simulink model "modelClosedLoop"  (R2019b)
settings: Solver=VariableStepAuto  StartTime=0.0  StopTime=Tsim  RelTol=1e-3
values from neighbouring files (symbols this model uses):
  vx = 2.0    (= 2)    [init_sim.m]
  X0 = zeros(7, 1)    [init_sim.m]
undefined symbols (not defined in the file or in its folder): Controlador, controllerGainsCurve, params, Ts_guidance, useCourse, userParameters, wps
settings Model: Creator=renan  LastModifiedBy=renan

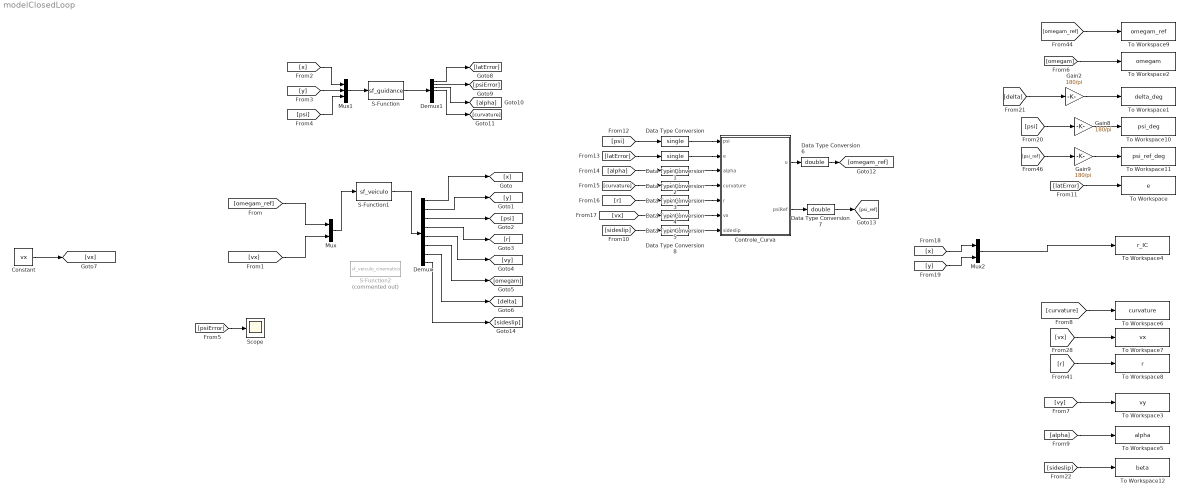
== system modelClosedLoop ==
  Constant : Constant  Value=vx
  Controle_Curva : Subsystem  TreatAsAtomicUnit=on
  Data Type Conversion{,1..5,8} (7 alike) : DataTypeConversion  OutDataTypeStr=single
  Data Type Conversion6 : DataTypeConversion  OutDataTypeStr=double
  Data Type Conversion7 : DataTypeConversion  OutDataTypeStr=double
  Demux : Demux  Outputs=8
  Demux1 : Demux  Outputs=7
  Gain2 : Gain  Gain=180/pi
  Gain8 : Gain  Gain=180/pi
  Gain9 : Gain  Gain=180/pi
  Mux : Mux  Inputs=2
  Mux1 : Mux  Inputs=3
  Mux2 : Mux  Inputs=2
  S-Function : S-Function  FunctionName=sf_guidance  Parameters=wps,Ts_guidance  SFunctionDeploymentMode=off  EnableBusSupport=off
  S-Function1 : S-Function  FunctionName=sf_veiculo  Parameters=X0,params  SFunctionDeploymentMode=off  EnableBusSupport=off
  S-Function2 : S-Function  Commented=on  FunctionName=sf_veiculo_cinematico  Parameters=X0,params  SFunctionDeploymentMode=off  EnableBusSupport=off
  Scope : Scope
  To Workspace : ToWorkspace  VariableName=e  SaveFormat=Structure With Time  SampleTime=0.01
  To Workspace1 : ToWorkspace  VariableName=delta_deg  SaveFormat=Structure With Time  SampleTime=0.01
  To Workspace10 : ToWorkspace  VariableName=psi_deg  SaveFormat=Structure With Time  SampleTime=0.01
  To Workspace11 : ToWorkspace  VariableName=psi_ref_deg  SaveFormat=Structure With Time  SampleTime=0.01
  To Workspace12 : ToWorkspace  VariableName=beta  SaveFormat=Structure With Time  SampleTime=0.01
  To Workspace2 : ToWorkspace  VariableName=omegam  SaveFormat=Structure With Time  SampleTime=0.01
  To Workspace3 : ToWorkspace  VariableName=vy  SaveFormat=Structure With Time  SampleTime=0.01
  To Workspace4 : ToWorkspace  VariableName=r_IC  SaveFormat=Structure With Time  SampleTime=0.01
  To Workspace5 : ToWorkspace  VariableName=alpha  SaveFormat=Structure With Time  SampleTime=0.01
  To Workspace6 : ToWorkspace  VariableName=curvature  SaveFormat=Structure With Time  SampleTime=0.01
  To Workspace7 : ToWorkspace  VariableName=vx  SaveFormat=Structure With Time  SampleTime=0.01
  To Workspace8 : ToWorkspace  VariableName=r  SaveFormat=Structure With Time  SampleTime=0.01
  To Workspace9 : ToWorkspace  VariableName=omegam_ref  SaveFormat=Structure With Time  SampleTime=0.01
  wires:
  Mux/1 -> S-Function1/1
  [omegam_ref] -> Mux/1
  [vx] -> Mux/2
  S-Function1/1 -> Demux/1
  Demux/1 -> [x]
  Demux/2 -> [y]
  Demux/3 -> [psi]
  Demux/4 -> [r]
  Demux/5 -> [vy]
  Demux/6 -> [omegam]
  Demux/7 -> [delta]
  Constant/1 -> [vx]
  [x] -> Mux1/1
  [y] -> Mux1/2
  Mux1/1 -> S-Function/1
  [psi] -> Mux1/3
  S-Function/1 -> Demux1/1
  Demux1/1 -> [latError]
  Demux1/2 -> [psiError]
  Demux1/3 -> [alpha]
  Demux1/4 -> [curvature]
  [latError] -> Data Type Conversion1/1
  [alpha] -> Data Type Conversion2/1
  [curvature] -> Data Type Conversion3/1
  [r] -> Data Type Conversion4/1
  [vx] -> Data Type Conversion5/1
  Controle_Curva/1(u) -> Data Type Conversion6/1
  Data Type Conversion/1 -> Controle_Curva/1(psi)
  Data Type Conversion1/1 -> Controle_Curva/2(e)
  Data Type Conversion2/1 -> Controle_Curva/3(alpha)
  Data Type Conversion3/1 -> Controle_Curva/4(curvature)
  Data Type Conversion4/1 -> Controle_Curva/5(r)
  Data Type Conversion5/1 -> Controle_Curva/6(vx)
  Data Type Conversion6/1 -> [omegam_ref]
  [curvature] -> To Workspace6/1
  Gain8/1 -> To Workspace10/1
  [latError] -> To Workspace/1
  [psi] -> Gain8/1
  Gain2/1 -> To Workspace1/1
  Gain9/1 -> To Workspace11/1
  [psi_ref] -> Gain9/1
  [omegam] -> To Workspace2/1
  [r] -> To Workspace8/1
  [omegam_ref] -> To Workspace9/1
  [vx] -> To Workspace7/1
  Mux2/1 -> To Workspace4/1
  [delta] -> Gain2/1
  Controle_Curva/2(psiRef) -> Data Type Conversion7/1
  Data Type Conversion7/1 -> [psi_ref]
  [x] -> Mux2/1
  [y] -> Mux2/2
  [psiError] -> Scope/1
  [vy] -> To Workspace3/1
  [alpha] -> To Workspace5/1
  Demux/8 -> [sideslip]
  [psi] -> Data Type Conversion/1
  [sideslip] -> Data Type Conversion8/1
  Data Type Conversion8/1 -> Controle_Curva/7(sideslip)
  [sideslip] -> To Workspace12/1

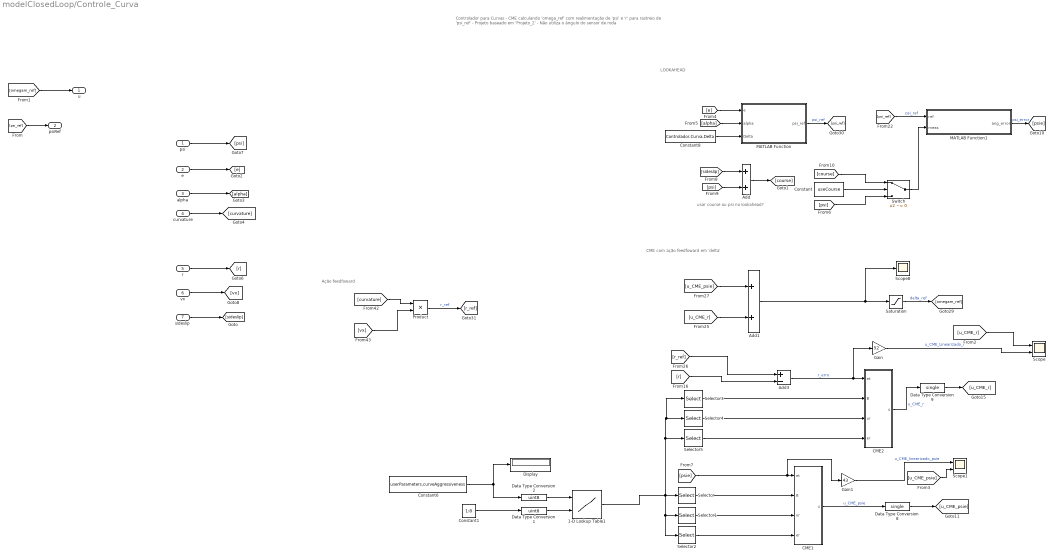
== system modelClosedLoop/Controle_Curva ==
  note: usar course ou psi no lookahead?
  note: Controlador para Curvas
      |
      | - CME calculando 'omega_ref' com realimentação de 'psi' e 'r' para rastreio de 'psi_ref'
      | - Projeto baseado em 'Projeto_2'
      | - Não utiliza o ângulo do sensor de roda
  note: LOOKAHEAD
  note: CME com ação feedfoward em 'delta'
  note: Ação feedfoward
  psi : Inport  OutDataTypeStr=single  PortDimensions=1
  e : Inport  Port=2  OutDataTypeStr=single  PortDimensions=1
  alpha : Inport  Port=3  OutDataTypeStr=single  PortDimensions=1
  curvature : Inport  Port=4  OutDataTypeStr=single  PortDimensions=1
  r : Inport  Port=5  OutDataTypeStr=single  PortDimensions=1
  vx : Inport  Port=6  OutDataTypeStr=single  PortDimensions=1
  sideslip : Inport  Port=7
  1-D Lookup Table1 : Lookup_n-D  BreakpointsForDimension1=uint8(1:7)  BreakpointsForDimension2=uint8(1:8)  IndexSearchMethod=Linear search  BeginIndexSearchUsingPreviousIndexResult=on  Table=controllerGainsCurve  ExtrapMethod=Clip  UseLastTableValue=on  InternalRulePriority=Speed  OutDataTypeStr=single  RndMeth=Simplest  InputSameDT=on
  Add : Sum
  Add1 : Sum
  Add3 : Sum  Inputs=+-
  CME1 : MATLAB Function  TreatAsAtomicUnit=on
  CME2 : MATLAB Function  TreatAsAtomicUnit=on
  Constant : Constant  Value=useCourse
  Constant1 : Constant  Value=1:8
  Constant6 : Constant  Value=userParameters.curveAggressiveness
  Constant8 : Constant  Value=Controlador.Curva.Delta  SampleTime=-1
  Data Type Conversion1 : DataTypeConversion  OutDataTypeStr=uint8
  Data Type Conversion2 : DataTypeConversion  OutDataTypeStr=uint8
  Data Type Conversion8 : DataTypeConversion  OutDataTypeStr=single
  Data Type Conversion9 : DataTypeConversion  OutDataTypeStr=single
  Display : Display
  Gain : Gain  Gain=52
  Gain1 : Gain  Gain=43
  MATLAB Function : MATLAB Function  TreatAsAtomicUnit=on
  MATLAB Function1 : MATLAB Function  TreatAsAtomicUnit=on
  Product : Product
  Saturation : Saturate  UpperLimit=Controlador.Curva.omegam_sat  LowerLimit=-Controlador.Curva.omegam_sat
  Scope : Scope  NumInputPorts=2
  Scope1 : Scope  NumInputPorts=2
  Scope8 : Scope
  Selector : Selector  InputPortWidth=8  IndexOptions=Index vector (dialog)  Indices=[2]  OutputSizes=1
  Selector1 : Selector  InputPortWidth=8  IndexOptions=Index vector (dialog)  Indices=[3 4]  OutputSizes=1
  Selector2 : Selector  InputPortWidth=8  IndexOptions=Index vector (dialog)  Indices=[1]  OutputSizes=1
  Selector3 : Selector  InputPortWidth=8  IndexOptions=Index vector (dialog)  Indices=[6]  OutputSizes=1
  Selector4 : Selector  InputPortWidth=8  IndexOptions=Index vector (dialog)  Indices=[7 8]  OutputSizes=1
  Selector5 : Selector  InputPortWidth=8  IndexOptions=Index vector (dialog)  Indices=[5]  OutputSizes=1
  Switch : Switch  Criteria=u2 ~= 0
  u : Outport
  psiRef : Outport  Port=2
  wires:
  [psi_ref] -> MATLAB Function1/1(ref)  "psi_ref"
  Constant8/1 -> MATLAB Function/3(Delta)
  MATLAB Function/1(psi_ref) -> [psi_ref]  "psi_ref"
  MATLAB Function1/1(ang_error) -> [psie]  "psi_error"
  [e] -> MATLAB Function/1(e)
  [alpha] -> MATLAB Function/2(alpha)
  Add1/1 -> Scope8/1, Saturation/1
  [u_CME_r] -> Add1/2
  CME2/1(u) -> Data Type Conversion9/1  "u_CME_r"
  CME1/1(u) -> Data Type Conversion8/1  "u_CME_psie"
  [r_ref] -> Add3/1
  [u_CME_psie] -> Add1/1
  [r] -> Add3/2
  Saturation/1 -> [omegam_ref]  "delta_ref"
  Product/1 -> [r_ref]  "r_ref"
  [curvature] -> Product/1
  [vx] -> Product/2
  psi/1 -> [psi]
  e/1 -> [e]
  alpha/1 -> [alpha]
  curvature/1 -> [curvature]
  r/1 -> [r]
  Add3/1 -> Gain/1, CME2/1(et)  "r_erro"
  [omegam_ref] -> u/1
  vx/1 -> [vx]
  [psie] -> CME1/1(et), Gain1/1
  Selector/1 -> CME1/2(B)
  Selector1/1 -> CME1/3(ur)
  Selector2/1 -> CME1/4(er)
  Selector3/1 -> CME2/2(B)
  Selector4/1 -> CME2/3(ur)
  Selector5/1 -> CME2/4(er)
  Data Type Conversion8/1 -> [u_CME_psie]
  Data Type Conversion9/1 -> [u_CME_r]
  Gain/1 -> Scope/2  "u_CME_Linearizado_r"
  Gain1/1 -> Scope1/1  "u_CME_linearizado_psie"
  Constant6/1 -> Display/1, Data Type Conversion2/1
  Constant1/1 -> Data Type Conversion1/1
  1-D Lookup Table1/1 -> Selector3/1, Selector4/1, Selector5/1, Selector2/1, Selector1/1, Selector/1
  Data Type Conversion2/1 -> 1-D Lookup Table1/1
  Data Type Conversion1/1 -> 1-D Lookup Table1/2
  [psi_ref] -> psiRef/1
  [u_CME_r] -> Scope/1
  [u_CME_psie] -> Scope1/2
  sideslip/1 -> [sideslip]
  [sideslip] -> Add/1
  [psi] -> Add/2
  Add/1 -> [course]
  Switch/1 -> MATLAB Function1/2(meas)
  Constant/1 -> Switch/2
  [course] -> Switch/1
  [psi] -> Switch/3

== matlab function modelClosedLoop/Controle_Curva/MATLAB Function ==
  data: e input; psi_ref output; alpha input; Delta input
function psi_ref = Lookahead(e, alpha, Delta)

psi_ref = alpha + atan(-e/Delta);

== matlab function modelClosedLoop/Controle_Curva/MATLAB Function1 ==
  data: ref input; ang_error output; meas input
% ref-meas
function ang_error = Angular_Error(ref, meas)

    ref = mod(ref, 2*pi);
    meas = mod(meas, 2*pi);
    
    if(meas > ref)
        if(abs(2*pi-meas+ref) < abs(ref-meas))
            ang_error = 2*pi-meas+ref;
        else
            ang_error = ref - meas;
        end
    elseif (meas < ref)
        if(abs(meas - ref) < abs(2*pi-ref+meas))
            ang_error = ref - meas;
        else
            ang_error = -(meas + 2*pi - ref);
        end
    else
        ang_error = single(0);
    end
end

== matlab function modelClosedLoop/Controle_Curva/CME1 ==
  data: u output size=1; et input size=1; B input size=1; ur input size=[2,1]; er input size=1
% et: erro (ref-meas)
% B: Parâmetro 3
% ur: Parâmetro 2 (batentes do controle)
% er: Parâmetro
function u = CME(et, B, ur, er)


umin = ur(1); umax = ur(2);
% Cálculo do erro
%et = yref - y;
e = et / er;
if e < -1, e = single(-1);  elseif e > 1, e = single(1); end
% Cálculo de u
if abs(e) == 1, ut = e; else ss = e - sign(e); ut = sign(ss) * (abs(ss) ^ (2 ^ -B) - 1); end
% Cálculo da saída
a = (umax - umin) / 2; u = a * (ut - 1) + umax;

end

== matlab function modelClosedLoop/Controle_Curva/CME2 ==
  data: u output size=1; et input size=1; B input size=1; ur input size=[2,1]; er input size=1
% et: erro (ref-meas)
% B: Parâmetro 3
% ur: Parâmetro 2 (batentes do controle)
% er: Parâmetro
function u = CME(et, B, ur, er)


umin = ur(1); umax = ur(2);
% Cálculo do erro
%et = yref - y;

e = et / er;

if e < -1
    e = single(-1);
elseif e > 1
    e = single(1);
end

% Cálculo de u
if abs(e) == 1
    ut = e;
else
    ss = e - sign(e);
    ut = sign(ss) * (abs(ss) ^ (2 ^ -B) - 1);
end

% Cálculo da saída
a = (umax - umin) / 2; u = a * (ut - 1) + umax;

end
